simulink library "ScienceStimHasomed"  (Simulink 6.2)
settings Model: LastModifiedBy=saunders

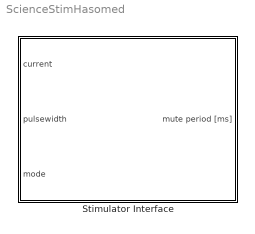
== system ScienceStimHasomed ==
  Stimulator Interface : Subsystem  mask(Stimulator Interface (RehaStim - Hasomed GmbH)){Ts=0.05, com_port=COM2, channelstim=[1 2], tsone=0, tstwo=5, channellf=[], nfactor=[]}
      mask prompts: Ts "Sample Time:"; com_port "Serial Port:"; channelstim "Channels to be Stimulated:"; tsone "Main Time in ms (only in steps of 0.5 ms):"; tstwo "Group Time in ms (only in steps of 0.5 ms):"; channellf "Low Frequency Channels:"; nfactor "Low Frequency Factor:"
      mask help:
      | Communication to the 8-channel RehaStim Stimulator (HASOMED GmbH) through the serial port.
      |
      | Sample Time:	  The sample time of the block (not neccessarily of the stimulation).
      | Serial Port:	  The serial port connected to the stimulator.
      | Channels:	  An array of channel numbers to be used (e.g. [1 2 5]).
      | Main Time:	  The stimulation period (set this to 0 for external triggering).
      | Group Time:	  The time between pulses in a group (doublet or triplet).
      | Low Freq Ch:	  A sub-set of the channels selected for low frequency.
      | Low Freq Fc:	  Stimulation is only every n times (n=factor).
      mask Help: eval('open(''SciencStimHasomed_Help.html'')')
      mask StyleString: edit,popup(COM1|COM2|COM3|COM4|COM5),edit,edit,edit,edit,edit
      mask Display:
      | image(imread('RehaStim_bg.jpg'), [0.05 0.15 0.9 0.6]);
      | image(imread('sciencestim_logo.png'), [0.95-0.4 0.03 0.4 0.15]);
      | image(imread('Hasomed_logo.bmp'), [0.95-0.6 0.95-0.2 0.6 0.2]);
      | port_label('input', 1, 'current');
      | port_label('input', 2, 'pulsewidth');
      | port_label('input', 3, 'mode');
      | port_label('output', 1, 'mute period [ms]');

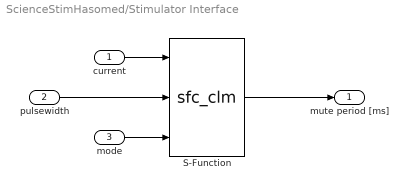
== system ScienceStimHasomed/Stimulator Interface ==
  current : Inport  Port=1  LatchInput=off
  pulsewidth : Inport  Port=2  LatchInput=off
  mode : Inport  Port=3  LatchInput=off
  S-Function : S-Function  FunctionName=sfc_clm  Parameters=Ts,com_port,channelstim,tsone,tstwo,0,channellf,nfactor
  mute period [ms] : Outport
  wires:
  S-Function/1 -> mute period [ms]/1
  mode/1 -> S-Function/3
  pulsewidth/1 -> S-Function/2
  current/1 -> S-Function/1
